simulink model "TOGGLER"  (R2022b)
settings: Solver=FixedStepDiscrete  StartTime=0  StopTime=duration  FixedStep=sample_time  RelTol=1e-3
values from neighbouring files (symbols this model uses):
  CTRL =     [TOGGLER_params.mat]
  CTRLSector =     [TOGGLER_params.mat]
  Greedy_Status = 1    [TOGGLER_params.mat]    (also in init_TOGGLER.m = logical(true))
  sample_time = 0.1    [TOGGLER_params.mat]
  WFC_1_Status = 1    [TOGGLER_params.mat]    (also in init_TOGGLER.m = logical(true))
  WFC_2_Status = 1    [TOGGLER_params.mat]    (also in init_TOGGLER.m = logical(true))
  WFC_3_Status = 1    [TOGGLER_params.mat]    (also in init_TOGGLER.m = logical(true))
undefined symbols (not defined in the file or in its folder): j
libraries: simulink x39, dspindex x14, dspstat3 x4, dspsigops x1
(part 1 of 2)
settings Model: Creator=Carlo_TUM  LastModifiedBy=Carlo_TUM
settings DataIOCC: LoadExternalInput=on  ReturnWorkspaceOutputs=off  ReturnWorkspaceOutputsName=off
settings OptimizationCC: DefaultParameterBehavior=Inlined  EnhancedBackFolding=on  PassReuseOutputArgsAs=Individual arguments  OptimizeBlockOrder=speed  DifferentSizesBufferReuse=on  OptimizationCustomize=off  EfficientTunableParamExpr=on
settings DebuggingCC: ParameterTunabilityLossMsg=error
settings SFSimCC: MATLABDynamicMemAlloc=off
settings RTWCC: Description=Embedded Coder  SystemTargetFile=ert.tlc  TemplateMakefile=ert_default_tmf
settings CodeAppCC: ForceParamTrailComments=on  IgnoreCustomStorageClasses=off  OperatorAnnotations=on  SimulinkDataObjDesc=on  SFDataObjDesc=on  InsertBlockDesc=on
settings ERTTargetCC: GenerateSampleERTMain=on  InlinedParameterPlacement=NonHierarchical  ERTCustomFileTemplate=example_file_process.tlc

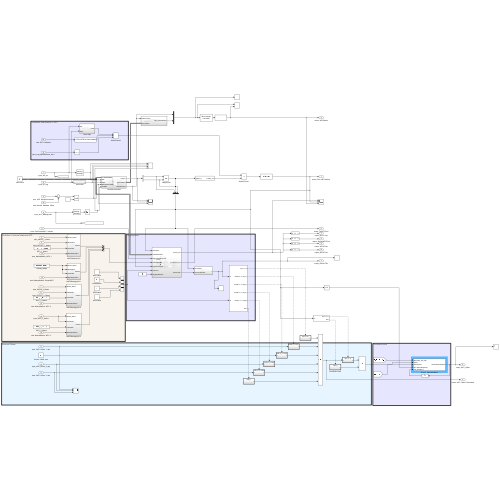
[thumbnail: Simulink's stored preview of the top-level diagram]
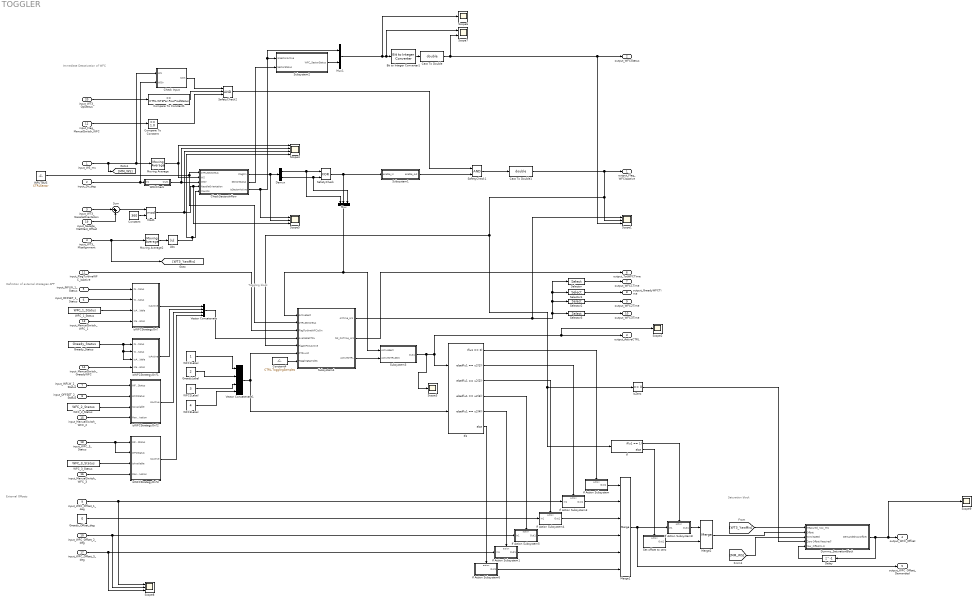
== system TOGGLER ==
  note: Definition of external strategies APP
  note: Toggling block
  note: External Offsets
  note: Saturation block
  note: Immediate Deactivation of WFC
  input_WS_ms : Inport  PortDimensions=1
  input_Dir_deg : Inport  Port=2  PortDimensions=1
  input_WT3_NacelleOrientation : Inport  Port=3  OutDataTypeStr=double  PortDimensions=1
  input_WT3_Misalignment : Inport  Port=4  OutDataTypeStr=double  PortDimensions=1
  input_INFLW_1_Status : Inport  Port=5  OutDataTypeStr=double
  input_OFFSET_1_Status : Inport  Port=6  OutDataTypeStr=double
  input_INFLW_2_Status : Inport  Port=7  OutDataTypeStr=double
  input_OFFSET_2_Status : Inport  Port=8
  input_WFC_Offset_1_deg : Inport  Port=9
  input_WFC_Offset_2_deg : Inport  Port=10
  input_FlagTurbineWFC_isActive : Inport  Port=11
  input_Flag_ManualSwitch_WFC : Inport  Port=12  PortDimensions=1
  input_ManualSwitch_WFC_1 : Inport  Port=13  PortDimensions=1
  input_ManualSwitch_GreedyWFC : Inport  Port=14  PortDimensions=1
  input_ManualSwitch_WFC_2 : Inport  Port=15  PortDimensions=1
  input_ManualSwitch_WFC_3 : Inport  Port=16  PortDimensions=1
  input_WFC_Offset_3_deg : Inport  Port=17  PortDimensions=1
  input_WFC_3_Status : Inport  Port=18  PortDimensions=1
  input_Nacelle_MetMast_Offset : Inport  Port=19  PortDimensions=1
  input_WT3_OpStatus : Inport  Port=20  PortDimensions=1
  Abs : Abs  SaturateOnIntegerOverflow=off
  Bit to Integer Converter1 : simulink/Logic and Bit Operations/Bit to Integer Converter  nbits=5  bitOrder=MSB first  signedOutputValues=Unsigned  outDtype=Inherit via internal rule  outDtypeSigned=Inherit via internal rule
      settings: LibrarySourceBlock=|
      | commutil2/Bit to Integer
      | Converter
  Cast To Double : DataTypeConversion  OutDataTypeStr=double  SaturateOnIntegerOverflow=off  RndMeth=Floor
  Cast To Double1 : DataTypeConversion  OutDataTypeStr=double  SaturateOnIntegerOverflow=off  RndMeth=Floor
  Check Input : Subsystem
  CheckSectorsInflow : Subsystem
  Compare To Constant : simulink/Logic and Bit Operations/Compare To Constant  relop===  const=1.0  OutDataTypeStr=boolean
  Compare To Constant1 : simulink/Logic and Bit Operations/Compare To Constant  relop===  const=CTRL.WT3Par.PowProdStatus  OutDataTypeStr=boolean
  Constant : Constant  Value=360
  Constant4 : Constant  Value=CTRL.TogglingSamples
  Delay : Delay  DelayLength=1  InitialCondition=0
  Demux : Demux  Outputs=2
  Dummy_SaturationBlock : Subsystem
  GreedyLabel : Constant  Value=2
  Greedy_Offset_deg : Constant  Value=0  OutDataTypeStr=Inherit: Inherit via back propagation
  Greedy_Status : Constant  Value=Greedy_Status
  INPUTBUS : Constant  Value=CTRLSector  VectorParams1D=off  OutDataTypeStr=Bus: CTRLSector_Bus
  If : If  IfExpression=u1 == 1
  If Action Subsystem : Subsystem  TreatAsAtomicUnit=on
  If Action Subsystem1 : Subsystem  TreatAsAtomicUnit=on
  If Action Subsystem3 : Subsystem  TreatAsAtomicUnit=on
  If Action Subsystem4 : Subsystem  TreatAsAtomicUnit=on
  If Action Subsystem5 : Subsystem  TreatAsAtomicUnit=on
  If Action Subsystem6 : Subsystem  TreatAsAtomicUnit=on
  If Action Subsystem8 : Subsystem  TreatAsAtomicUnit=on
  If3 : If  NumInputs=2  IfExpression=u1 == 0  ElseIfExpressions=u1 == u2(1) , u1 == u2(2) , u1 == u2(3) , u1 == u2(4)
  IsZero : simulink/Logic and Bit Operations/Compare To Zero  relop===  OutDataTypeStr=boolean
  Merge1 : Merge  Inputs=6
  Merge2 : Merge
  Mod1 : Math  Operator=mod  SignedPower=on
  Moving Average : dspstat3/Moving Average  Method=Sliding window  ForgettingFactorPort=off  SpecifyWindowLength=on  WindowLength=CTRL.MovAvWS  OverlapLength=CTRL.MovAvWS - 1  AllowArbitraryInputLength=off  ForgettingFactor=0.9  SimulateUsing=Code generation
  Moving Average2 : dspstat3/Moving Average  Method=Sliding window  ForgettingFactorPort=off  SpecifyWindowLength=on  WindowLength=CTRL.MovAvWMisalignment  OverlapLength=CTRL.MovAvWMisalignment - 1  AllowArbitraryInputLength=off  ForgettingFactor=0.9  SimulateUsing=Code generation
  Mux : Mux  Inputs=3
  Mux1 : Mux  Inputs=2
  SafetyCheck : Logic  Operator=XOR  AllPortsSameDT=off  OutDataTypeStr=boolean
  SafetyCheck1 : Logic  AllPortsSameDT=off  OutDataTypeStr=boolean
  SafetyCheck2 : Logic  Inputs=3  AllPortsSameDT=off  OutDataTypeStr=boolean
  Scope1 : Scope  NumInputPorts=3
  Scope{2..3,6,9} (4 alike) : Scope
  Scope4 : Scope  NumInputPorts=4
  Scope5 : Scope  NumInputPorts=3
  Scope7 : Scope  NumInputPorts=2
  Scope8 : Scope  NumInputPorts=3
  Selector : Selector  InputPortWidth=4  IndexOptions=Index vector (dialog)  Indices=[1]  OutputSizes=1
  Selector1 : Selector  InputPortWidth=4  IndexOptions=Index vector (dialog)  Indices=[2]  OutputSizes=1
  Selector2 : Selector  InputPortWidth=4  IndexOptions=Index vector (dialog)  Indices=[3]  OutputSizes=1
  Selector3 : Selector  InputPortWidth=4  IndexOptions=Index vector (dialog)  Indices=[4]  OutputSizes=1
  Set offset to zero : Subsystem  TreatAsAtomicUnit=on
  Subsystem1 : Subsystem  mask(Signal holding){wait_time=CTRL.InflowChecks_WaitTime, sampling_time=sample_time, selection=off}
      mask prompts: wait_time "Wait time [s]"; sampling_time "Sampling time [s]"; selection "Instant disabling"
      mask help:
      | The block prevents fast switching of the input signal. After the input is changed, it waits for the defined time before changing the output, if the input doesn't change within this period, the output is switched.
      | The option "Instant disabling" only enforces waiting time on rising edge, but always allows the signal to go to zero.
      | Ask Vlaho for help.
      mask init:
      | Counter = wait_time/sampling_time;
      mask Help:
      | No documentation, ask Vlaho for help. ;)
      | 22 Nov 2020
  Subsystem2 : Subsystem
  Subsystem3 : Subsystem
  Subsystem4 : Subsystem
  Sum : Sum  Inputs=|++
  Vector Concatenate : Concatenate  NumInputs=4
  Vector Concatenate1 : Concatenate  NumInputs=4
  WDirCheck : Subsystem
  WFC1Label : Constant
  WFC2Label : Constant  Value=3
  WFC3Label : Constant  Value=4
  WFC_1_Status : Constant  Value=WFC_1_Status
  WFC_2_Status : Constant  Value=WFC_2_Status
  WFC_3_Status : Constant  Value=WFC_3_Status
  isWFCStrategyOn? : Subsystem
  isWFCStrategyOn?1 : Subsystem
  isWFCStrategyOn?2 : Subsystem
  isWFCStrategyOn?3 : Subsystem
  output_Flag_WFCIsActive : Outport  VectorParamsAs1DForOutWhenUnconnected=off
  output_WFCStatus : Outport  Port=2  VectorParamsAs1DForOutWhenUnconnected=off
  output_ActiveCTRL : Outport  Port=3  VectorParamsAs1DForOutWhenUnconnected=off
  output_WFC_Offset : Outport  Port=4  VectorParamsAs1DForOutWhenUnconnected=off
  output_WFC_Offset_Demanded : Outport  Port=5  VectorParamsAs1DForOutWhenUnconnected=off
  output_TotWFCTime : Outport  Port=6  VectorParamsAs1DForOutWhenUnconnected=off
  output_WFC1Time : Outport  Port=7  VectorParamsAs1DForOutWhenUnconnected=off
  output_GreedyWFCTime : Outport  Port=8  VectorParamsAs1DForOutWhenUnconnected=off
  output_WFC2Time : Outport  Port=9  VectorParamsAs1DForOutWhenUnconnected=off
  output_WFC3Time : Outport  Port=10  VectorParamsAs1DForOutWhenUnconnected=off
  wires:
  SafetyCheck1/1 -> Cast To Double1/1
  Subsystem4/3(ActiveCTRL) -> Subsystem3/2(ActiveCTRLSect)
  If3/1 -> If Action Subsystem/Action
  Abs/1 -> CheckSectorsInflow/5(YawMis), Scope4/4
  CheckSectorsInflow/2(SectorStatus) -> Subsystem2/2(SectorStatus)
  input_ManualSwitch_GreedyWFC/1 -> isWFCStrategyOn?1/4(ManualActivation)
  input_Dir_deg/1 -> Check Input/2(WDir), WDirCheck/1(In1)
  Selector3/1 -> output_WFC3Time/1
  isWFCStrategyOn?2/1(isActive) -> Vector Concatenate/3
  Vector Concatenate1/1 -> Subsystem4/6(CTRLList), If3/2
  input_ManualSwitch_WFC_1/1 -> isWFCStrategyOn?/4(ManualActivation)
  Demux/1 -> Mux/1, SafetyCheck/1
  Selector1/1 -> output_GreedyWFCTime/1
  Dummy_SaturationBlock/1(DemandedYawOffset) -> Delay/1, Scope9/1, output_WFC_Offset/1
  input_WS_ms/1 -> Check Input/1(WS), Moving Average/1, [MM_WS]
  input_Nacelle_MetMast_Offset/1 -> Sum/2
  Check Input/1(IsOK) -> SafetyCheck2/1
  WFC_1_Status/1 -> isWFCStrategyOn?/3(isAvailable)
  input_INFLW_2_Status/1 -> isWFCStrategyOn?2/1(INFLW_Status)
  input_Flag_ManualSwitch_WFC/1 -> Compare To Constant/1
  isWFCStrategyOn?/1(isActive) -> Vector Concatenate/1
  SafetyCheck/1 -> Subsystem1/1(enable_in), Mux/2
  Compare To Constant1/1 -> SafetyCheck2/2
  input_WT3_OpStatus/1 -> Compare To Constant1/1
  If Action Subsystem1/1(Out1) -> Merge1/5
  If Action Subsystem5/1(Out1) -> Merge1/4
  [WT3_YawMis] -> Dummy_SaturationBlock/1(Measured_Yaw_Mis)
  input_WT3_Misalignment/1 -> [WT3_YawMis], Moving Average2/1
  input_WFC_3_Status/1 -> isWFCStrategyOn?3/2(WFCStatus), isWFCStrategyOn?3/1(INFLW_Status)
  WFC_3_Status/1 -> isWFCStrategyOn?3/3(isAvailable)
  Constant/1 -> Mod1/2
  isWFCStrategyOn?3/1(isActive) -> Vector Concatenate/4
  input_WFC_Offset_1_deg/1 -> Scope8/1, If Action Subsystem3/1(In1)
  Delay/1 -> Dummy_SaturationBlock/5(Yaw_Offset(k-1))
  WFC3Label/1 -> Vector Concatenate1/4
  If3/5 -> If Action Subsystem1/Action
  CheckSectorsInflow/3(isSectorActive) -> Scope5/1, Mux1/1, Subsystem2/1(isSectorActive)
  Greedy_Status/1 -> isWFCStrategyOn?1/2(WFCStatus), isWFCStrategyOn?1/3(isAvailable), isWFCStrategyOn?1/1(INFLW_Status)
  Constant4/1 -> Subsystem4/7(TogglingSamples)
  If3/3 -> If Action Subsystem4/Action
  Cast To Double1/1 -> IsZero/1, If/1, Subsystem4/5(FlagWFCIsActive), Scope1/2, output_Flag_WFCIsActive/1
  Subsystem4/2(tot_OnTime_Hrs) -> output_TotWFCTime/1
  Subsystem4/1(onTime_Hrs) -> Scope1/1, Selector3/1, Selector/1, Selector1/1, Selector2/1
  isWFCStrategyOn?1/1(isActive) -> Vector Concatenate/2
  If Action Subsystem4/1(Out1) -> Merge1/3
  input_ManualSwitch_WFC_2/1 -> isWFCStrategyOn?2/4(ManualActivation)
  input_FlagTurbineWFC_isActive/1 -> Subsystem4/3(FlagTurbineWFCIsOn)
  Vector Concatenate/1 -> Subsystem4/4(AvailableCTRL)
  Selector2/1 -> output_WFC2Time/1
  If Action Subsystem8/1(Out1) -> Merge2/1
  GreedyLabel/1 -> Vector Concatenate1/2
  WFC_2_Status/1 -> isWFCStrategyOn?2/3(isAvailable)
  SafetyCheck2/1 -> SafetyCheck1/1
  input_ManualSwitch_WFC_3/1 -> isWFCStrategyOn?3/4(ManualActivation)
  input_OFFSET_1_Status/1 -> isWFCStrategyOn?/2(WFCStatus)
  Subsystem3/1(Out1) -> Scope3/1, output_ActiveCTRL/1, Scope2/1, If3/1
  INPUTBUS/1 -> Subsystem4/2(CTRLSectorBus), CheckSectorsInflow/1(CTRLSectorBus)
  Merge1/1 -> output_WFC_Offset_Demanded/1, If Action Subsystem8/1(In1)
  IsZero/1 -> Dummy_SaturationBlock/4(Zero Offset Required?)
  Mod1/1 -> Scope5/3, CheckSectorsInflow/4(NacelleOrientation), Scope4/3
  input_OFFSET_2_Status/1 -> isWFCStrategyOn?2/2(WFCStatus)
  input_WFC_Offset_3_deg/1 -> Scope8/3, If Action Subsystem1/1(In1)
  input_WFC_Offset_2_deg/1 -> Scope8/2, If Action Subsystem5/1(In1)
  Moving Average/1 -> CheckSectorsInflow/2(WS), Scope4/1
  Mux1/1 -> Scope6/1, Scope7/1, Bit to Integer Converter1/1
  WDirCheck/1(Out1) -> Scope4/2, CheckSectorsInflow/3(WDir)
  input_WT3_NacelleOrientation/1 -> Sum/1
  Merge2/1 -> Dummy_SaturationBlock/2(Offset)
  Mux/1 -> Subsystem3/1(ActiveSect), Subsystem4/1(ActiveSect)
  Cast To Double/1 -> Scope7/2, Scope1/3, output_WFCStatus/1
  CheckSectorsInflow/1(FlagOn) -> Scope5/2, Demux/1
  Sum/1 -> Mod1/1
  Bit to Integer Converter1/1 -> Cast To Double/1
  [MM_WS] -> Dummy_SaturationBlock/3(Wind Speed)
  input_INFLW_1_Status/1 -> isWFCStrategyOn?/1(INFLW_Status)
  Selector/1 -> output_WFC1Time/1
  WFC2Label/1 -> Vector Concatenate1/3
  Subsystem1/1(enable_out) -> SafetyCheck1/2
  Demux/2 -> Mux/3, SafetyCheck/2
  If3/2 -> If Action Subsystem3/Action
  If/2 -> Set offset to zero/Action
  WFC1Label/1 -> Vector Concatenate1/1
  Moving Average2/1 -> Abs/1
  Subsystem2/1(WFC_SectorStatus) -> Mux1/2
  Set offset to zero/1(Out1) -> Merge2/2
  Compare To Constant/1 -> SafetyCheck2/3
  If3/6 -> If Action Subsystem6/Action
  If3/4 -> If Action Subsystem5/Action
  Greedy_Offset_deg/1 -> If Action Subsystem4/1(In1)
  If Action Subsystem/1(Out1) -> Merge1/1
  If Action Subsystem6/1(Out1) -> Merge1/6
  If Action Subsystem3/1(Out1) -> Merge1/2
  If/1 -> If Action Subsystem8/Action

== system TOGGLER/Check Input ==
  WS : Inport
  WDir : Inport  Port=2
  Constant2 : Constant  Value=CTRL.InputCheck.StartupTimeSamples
  Logical Operator : Logic  Operator=OR  AllPortsSameDT=off  OutDataTypeStr=boolean
  NOT : Logic  Operator=NOT  IconShape=distinctive  AllPortsSameDT=off  OutDataTypeStr=boolean
  Scope9 : Scope  NumInputPorts=2
  Subsystem5 : Subsystem
  Subsystem6 : Subsystem
  Terminator : Terminator
  Terminator1 : Terminator
  IsOK : Outport  VectorParamsAs1DForOutWhenUnconnected=off
  wires:
  Subsystem6/1(Var) -> Terminator/1
  Subsystem5/1(Var) -> Terminator1/1
  Constant2/1 -> Subsystem6/2(StartupTimeSamples), Subsystem5/2(StartupTimeSamples)
  WS/1 -> Subsystem6/1(InVar)
  Subsystem6/2(ErrorFlag) -> Logical Operator/1, Scope9/1
  Subsystem5/2(ErrorFlag) -> Logical Operator/2, Scope9/2
  WDir/1 -> Subsystem5/1(InVar)
  Logical Operator/1 -> NOT/1
  NOT/1 -> IsOK/1

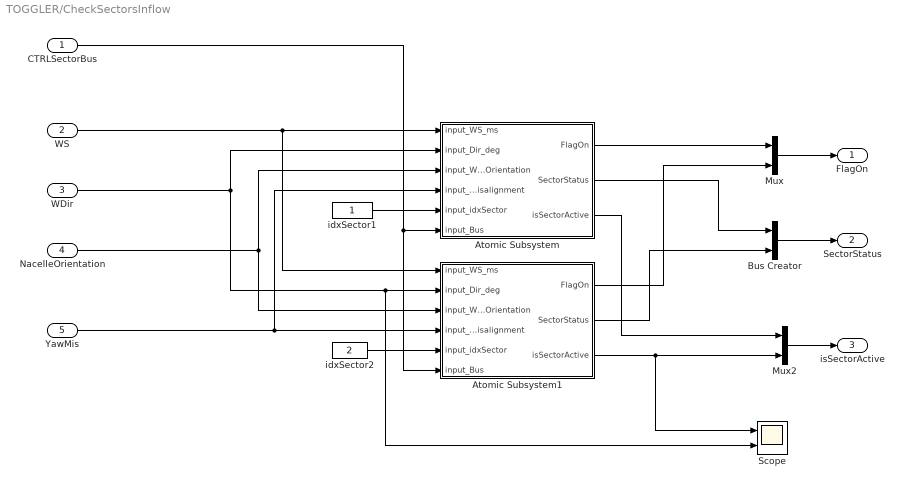
== system TOGGLER/CheckSectorsInflow ==
  CTRLSectorBus : Inport  OutDataTypeStr=Bus: CTRLSector_Bus
  WS : Inport  Port=2
  WDir : Inport  Port=3
  NacelleOrientation : Inport  Port=4
  YawMis : Inport  Port=5
  Atomic Subsystem : Subsystem  TreatAsAtomicUnit=on
  Atomic Subsystem1 : Subsystem  TreatAsAtomicUnit=on
  Bus Creator : BusCreator  Inputs=2
  Mux : Mux  Inputs=2
  Mux2 : Mux  Inputs=2
  Scope : Scope  NumInputPorts=2
  idxSector1 : Constant
  idxSector2 : Constant  Value=2
  FlagOn : Outport  VectorParamsAs1DForOutWhenUnconnected=off
  SectorStatus : Outport  Port=2  VectorParamsAs1DForOutWhenUnconnected=off
  isSectorActive : Outport  Port=3  VectorParamsAs1DForOutWhenUnconnected=off
  wires:
  Atomic Subsystem1/1(FlagOn) -> Mux/2
  idxSector1/1 -> Atomic Subsystem/5(input_idxSector)
  idxSector2/1 -> Atomic Subsystem1/5(input_idxSector)
  YawMis/1 -> Atomic Subsystem/4(input_WT3_Misalignment), Atomic Subsystem1/4(input_WT3_Misalignment)
  WS/1 -> Atomic Subsystem1/1(input_WS_ms), Atomic Subsystem/1(input_WS_ms)
  NacelleOrientation/1 -> Atomic Subsystem/3(input_WT3_NacelleOrientation), Atomic Subsystem1/3(input_WT3_NacelleOrientation)
  CTRLSectorBus/1 -> Atomic Subsystem1/6(input_Bus), Atomic Subsystem/6(input_Bus)
  WDir/1 -> Atomic Subsystem/2(input_Dir_deg), Scope/2, Atomic Subsystem1/2(input_Dir_deg)
  Atomic Subsystem/2(SectorStatus) -> Bus Creator/1
  Atomic Subsystem1/2(SectorStatus) -> Bus Creator/2
  Atomic Subsystem/3(isSectorActive) -> Mux2/1
  Atomic Subsystem1/3(isSectorActive) -> Scope/1, Mux2/2
  Atomic Subsystem/1(FlagOn) -> Mux/1
  Mux/1 -> FlagOn/1
  Bus Creator/1 -> SectorStatus/1
  Mux2/1 -> isSectorActive/1

== system TOGGLER/Dummy_SaturationBlock ==
  note: This is a dummy saturation block. In a real case, this block should include the actual control logic of the WT to prevent unwanted shut down during WFC
  Measured_Yaw_Mis : Inport
  Offset : Inport  Port=2
  Wind Speed : Inport  Port=3
  Zero Offset Required? : Inport  Port=4
  Yaw_Offset(k-1) : Inport  Port=5
  Saturation : Saturate  UpperLimit=CTRL.SatBlock.WFC_OffsetRange(2)  LowerLimit=CTRL.SatBlock.WFC_OffsetRange(1)
  Terminator{,1..2,4} (4 alike) : Terminator
  DemandedYawOffset : Outport  PortDimensions=1
  wires:
  Offset/1 -> Saturation/1
  Saturation/1 -> DemandedYawOffset/1
  Wind Speed/1 -> Terminator1/1
  Zero Offset Required?/1 -> Terminator/1
  Yaw_Offset(k-1)/1 -> Terminator2/1
  Measured_Yaw_Mis/1 -> Terminator4/1

== system TOGGLER/If Action Subsystem ==
  Action Port : ActionPort  ActionPortLabel=if(u1 == 0)
  Zero : Constant  Value=0  OutDataTypeStr=Inherit: Inherit via back propagation
  Out1 : Outport  VectorParamsAs1DForOutWhenUnconnected=off
  wires:
  Zero/1 -> Out1/1

== system TOGGLER/If Action Subsystem1 ==
  In1 : Inport
  Action Port : ActionPort  ActionPortLabel=elseif( u1 == u2(4))
  Out1 : Outport  VectorParamsAs1DForOutWhenUnconnected=off
  wires:
  In1/1 -> Out1/1

== system TOGGLER/If Action Subsystem3 ==
  In1 : Inport
  Action Port : ActionPort  ActionPortLabel=elseif(u1 == u2(1) )
  Out1 : Outport  VectorParamsAs1DForOutWhenUnconnected=off
  wires:
  In1/1 -> Out1/1

== system TOGGLER/If Action Subsystem4 ==
  In1 : Inport
  Action Port : ActionPort  ActionPortLabel=elseif( u1 == u2(2) )
  Out1 : Outport  VectorParamsAs1DForOutWhenUnconnected=off
  wires:
  In1/1 -> Out1/1

== system TOGGLER/If Action Subsystem5 ==
  In1 : Inport
  Action Port : ActionPort  ActionPortLabel=elseif( u1 == u2(3) )
  Out1 : Outport  VectorParamsAs1DForOutWhenUnconnected=off
  wires:
  In1/1 -> Out1/1

== system TOGGLER/If Action Subsystem6 ==
  Action Port : ActionPort  ActionPortLabel=else
  Zero : Constant  Value=0  OutDataTypeStr=Inherit: Inherit via back propagation
  Out1 : Outport  VectorParamsAs1DForOutWhenUnconnected=off
  wires:
  Zero/1 -> Out1/1

== system TOGGLER/If Action Subsystem8 ==
  In1 : Inport
  Action Port : ActionPort  ActionPortLabel=if(u1 == 1)
  Out1 : Outport  VectorParamsAs1DForOutWhenUnconnected=off
  wires:
  In1/1 -> Out1/1

== system TOGGLER/Set offset to zero ==
  Action Port : ActionPort  ActionPortLabel=else
  Zero : Constant  Value=0  OutDataTypeStr=Inherit: Inherit via back propagation
  Out1 : Outport  VectorParamsAs1DForOutWhenUnconnected=off
  wires:
  Zero/1 -> Out1/1

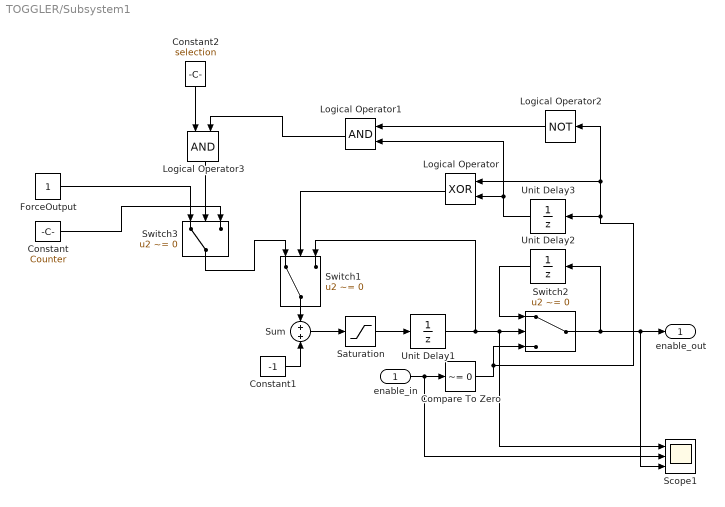
== system TOGGLER/Subsystem1 ==
  enable_in : Inport
  Compare To Zero : simulink/Logic and Bit Operations/Compare To Zero  relop=~=  OutDataTypeStr=boolean
  Constant : Constant  Value=Counter
  Constant1 : Constant  Value=-1
  Constant2 : Constant  Value=selection
  ForceOutput : Constant  OutDataTypeStr=Inherit: Inherit via back propagation
  Logical Operator : Logic  Operator=XOR  AllPortsSameDT=off  OutDataTypeStr=boolean
  Logical Operator1 : Logic  AllPortsSameDT=off  OutDataTypeStr=boolean
  Logical Operator2 : Logic  Operator=NOT  AllPortsSameDT=off  OutDataTypeStr=boolean
  Logical Operator3 : Logic  AllPortsSameDT=off  OutDataTypeStr=boolean
  Saturation : Saturate  UpperLimit=inf  LowerLimit=-inf
  Scope1 : Scope  NumInputPorts=3
  Sum : Sum
  Switch1 : Switch  Criteria=u2 ~= 0  SaturateOnIntegerOverflow=off  InputSameDT=off
  Switch2 : Switch  Criteria=u2 ~= 0  SaturateOnIntegerOverflow=off  InputSameDT=off
  Switch3 : Switch  Criteria=u2 ~= 0  SaturateOnIntegerOverflow=off  InputSameDT=off
  Unit Delay1 : UnitDelay  SampleTime=sampling_time  HasFrameUpgradeWarning=on
  Unit Delay2 : UnitDelay  SampleTime=sampling_time  HasFrameUpgradeWarning=on
  Unit Delay3 : UnitDelay  SampleTime=sampling_time  HasFrameUpgradeWarning=on
  enable_out : Outport
  wires:
  Saturation/1 -> Unit Delay1/1
  Unit Delay2/1 -> Switch2/1
  Switch2/1 -> Scope1/3, enable_out/1, Unit Delay2/1
  Sum/1 -> Saturation/1
  Switch1/1 -> Sum/1
  Constant1/1 -> Sum/2
  Constant/1 -> Switch3/3
  Logical Operator/1 -> Switch1/2
  enable_in/1 -> Scope1/2, Compare To Zero/1
  Logical Operator2/1 -> Logical Operator1/1
  Logical Operator1/1 -> Logical Operator3/2
  Compare To Zero/1 -> Switch2/3, Unit Delay3/1, Logical Operator/1, Logical Operator2/1
  Unit Delay3/1 -> Logical Operator/2, Logical Operator1/2
  Unit Delay1/1 -> Switch1/3, Scope1/1, Switch2/2
  Constant2/1 -> Logical Operator3/1
  ForceOutput/1 -> Switch3/1
  Switch3/1 -> Switch1/1
  Logical Operator3/1 -> Switch3/2

== system TOGGLER/Subsystem2 ==
  isSectorActive : Inport
  SectorStatus : Inport  Port=2
  Bus Selector : BusSelector  OutputSignals=signal1,signal2
  Demux : Demux  Outputs=2
  Enabled Subsystem : Subsystem  TreatAsAtomicUnit=on
  Enabled Subsystem1 : Subsystem  TreatAsAtomicUnit=on
  Gain : Gain  Gain=0
  Logical Operator : Logic  Operator=XOR  AllPortsSameDT=off  OutDataTypeStr=boolean
  Merge3 : Merge
  Switch : Switch  Criteria=u2 ~= 0  SaturateOnIntegerOverflow=off  InputSameDT=off
  WFC_SectorStatus : Outport  VectorParamsAs1DForOutWhenUnconnected=off
  wires:
  Demux/1 -> Logical Operator/1, Enabled Subsystem/Enable
  Logical Operator/1 -> Switch/2
  Bus Selector/2 -> Enabled Subsystem1/1(In1)  "<signal2>"
  Enabled Subsystem/1(Out1) -> Merge3/1
  Gain/1 -> Switch/3
  Merge3/1 -> Switch/1
  Bus Selector/1 -> Gain/1, Enabled Subsystem/1(In1)  "<signal1>"
  Enabled Subsystem1/1(Out1) -> Merge3/2
  Demux/2 -> Logical Operator/2, Enabled Subsystem1/Enable
  SectorStatus/1 -> Bus Selector/1
  Switch/1 -> WFC_SectorStatus/1
  isSectorActive/1 -> Demux/1

== system TOGGLER/Subsystem3 ==
  ActiveSect : Inport
  ActiveCTRLSect : Inport  Port=2
  Demux1 : Demux  Outputs=3
  Demux2 : Demux  Outputs=2
  Enabled Subsystem : Subsystem  TreatAsAtomicUnit=on
  Enabled Subsystem1 : Subsystem  TreatAsAtomicUnit=on
  Enabled Subsystem2 : Subsystem  TreatAsAtomicUnit=on
  Enabled Subsystem3 : Subsystem  TreatAsAtomicUnit=on
  Merge : Merge  Inputs=3
  Subsystem : Subsystem
  Out1 : Outport  VectorParamsAs1DForOutWhenUnconnected=off
  wires:
  Demux2/2 -> Enabled Subsystem2/4(ActiveCTRL_S2), Enabled Subsystem1/1(In1)
  ActiveSect/1 -> Demux1/1
  Demux1/2 -> Subsystem/2(XOR)
  Subsystem/3(Off) -> Enabled Subsystem3/Enable
  Demux1/1 -> Subsystem/1(Sect1)
  Demux1/3 -> Subsystem/3(Sect2)
  ActiveCTRLSect/1 -> Demux2/1
  Subsystem/2(Sector2_Flag) -> Enabled Subsystem1/Enable, Enabled Subsystem2/2(Sector2_Flag)
  Subsystem/1(Sector1_Flag) -> Enabled Subsystem/Enable, Enabled Subsystem2/1(Sector1_Flag)
  Demux2/1 -> Enabled Subsystem2/3(ActiveCTRL_S1), Enabled Subsystem/1(In1)
  Enabled Subsystem/1(Out1) -> Merge/2
  Enabled Subsystem1/1(Out1) -> Merge/3
  Enabled Subsystem2/1(Out1) -> Enabled Subsystem3/1(In1)
  Merge/1 -> Out1/1
  Enabled Subsystem3/1(Out1) -> Merge/1

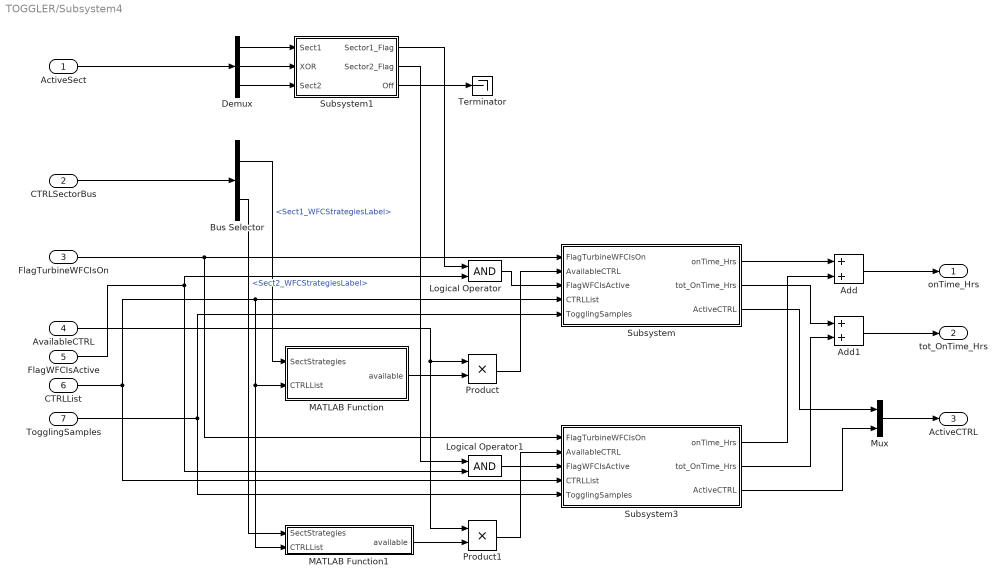
== system TOGGLER/Subsystem4 ==
  ActiveSect : Inport
  CTRLSectorBus : Inport  Port=2  OutDataTypeStr=Bus: CTRLSector_Bus
  FlagTurbineWFCIsOn : Inport  Port=3
  AvailableCTRL : Inport  Port=4
  FlagWFCIsActive : Inport  Port=5
  CTRLList : Inport  Port=6
  TogglingSamples : Inport  Port=7
  Add : Sum
  Add1 : Sum
  Bus Selector : BusSelector  OutputSignals=Sect1_WFCStrategiesLabel,Sect2_WFCStrategiesLabel
  Demux : Demux  Outputs=3
  Logical Operator : Logic  AllPortsSameDT=off  OutDataTypeStr=boolean
  Logical Operator1 : Logic  AllPortsSameDT=off  OutDataTypeStr=boolean
  MATLAB Function : MATLAB Function  TreatAsAtomicUnit=on
  MATLAB Function1 : MATLAB Function  TreatAsAtomicUnit=on
  Mux : Mux  Inputs=2
  Product : Product
  Product1 : Product
  Subsystem : Subsystem
  Subsystem1 : Subsystem
  Subsystem3 : Subsystem
  Terminator : Terminator
  onTime_Hrs : Outport  VectorParamsAs1DForOutWhenUnconnected=off
  tot_OnTime_Hrs : Outport  Port=2  VectorParamsAs1DForOutWhenUnconnected=off
  ActiveCTRL : Outport  Port=3  VectorParamsAs1DForOutWhenUnconnected=off
  wires:
  CTRLSectorBus/1 -> Bus Selector/1
  FlagTurbineWFCIsOn/1 -> Subsystem3/1(FlagTurbineWFCIsOn), Subsystem/1(FlagTurbineWFCIsOn)
  FlagWFCIsActive/1 -> Logical Operator1/2, Logical Operator/2
  CTRLList/1 -> Subsystem3/4(CTRLList), MATLAB Function1/2(CTRLList), MATLAB Function/2(CTRLList), Subsystem/4(CTRLList)
  TogglingSamples/1 -> Subsystem3/5(TogglingSamples), Subsystem/5(TogglingSamples)
  Bus Selector/1 -> MATLAB Function/1(SectStrategies)  "<Sect1_WFCStrategiesLabel>"
  MATLAB Function/1(available) -> Product/2
  Bus Selector/2 -> MATLAB Function1/1(SectStrategies)  "<Sect2_WFCStrategiesLabel>"
  MATLAB Function1/1(available) -> Product1/2
  AvailableCTRL/1 -> Product1/1, Product/1
  Product/1 -> Subsystem/2(AvailableCTRL)
  Product1/1 -> Subsystem3/2(AvailableCTRL)
  Subsystem/1(onTime_Hrs) -> Add/1
  Subsystem3/1(onTime_Hrs) -> Add/2
  Subsystem/2(tot_OnTime_Hrs) -> Add1/1
  Subsystem3/2(tot_OnTime_Hrs) -> Add1/2
  Add/1 -> onTime_Hrs/1
  Add1/1 -> tot_OnTime_Hrs/1
  Subsystem/3(ActiveCTRL) -> Mux/1
  Subsystem3/3(ActiveCTRL) -> Mux/2
  Mux/1 -> ActiveCTRL/1
  ActiveSect/1 -> Demux/1
  Demux/1 -> Subsystem1/1(Sect1)
  Demux/2 -> Subsystem1/2(XOR)
  Demux/3 -> Subsystem1/3(Sect2)
  Subsystem1/1(Sector1_Flag) -> Logical Operator/1
  Logical Operator/1 -> Subsystem/3(FlagWFCIsActive)
  Subsystem1/2(Sector2_Flag) -> Logical Operator1/1
  Logical Operator1/1 -> Subsystem3/3(FlagWFCIsActive)
  Subsystem1/3(Off) -> Terminator/1

== system TOGGLER/WDirCheck ==
  In1 : Inport
  Compare To Constant : simulink/Logic and Bit Operations/Compare To Constant  relop=>=  const=600.0  OutDataTypeStr=boolean
  Delay : Delay  DelayLength=1  InitialCondition=0
  Ground : Ground
  Sample and Hold : dspsigops/Sample and Hold  trig=Rising edge  initCond=0  latchinput=off
  Scope : Scope  NumInputPorts=3
  Subsystem5 : Subsystem  mask(Moving average & standard deviation for angles){filt_T=CTRL.MovAvWDir*sample_time, filt_wait=CTRL.MovAvWDir*sample_time, sample_time=sample_time}
      mask prompts: filt_T "Window duration"; filt_wait "Waiting time before providing output"; sample_time "Sample time"
      mask help:
      | Computes moving average and standard deviation for angular values in degrees over a time window. All parameters are expressed in seconds.
      | Ask Vlaho for details.
      | 25 Nov 2020
      mask init:
      | N_filt = ceil(filt_T / sample_time);
      | if N_filt<1, N_filt = 1; end
      | lower_limit = ceil(filt_wait / sample_time);
      | if lower_limit<2, lower_limit = 2; end
      mask Help: No help provided, ask Vlaho for details. ;)
  Switch : Switch  Criteria=u2 ~= 0  SaturateOnIntegerOverflow=off  InputSameDT=off
  Terminator : Terminator
  Terminator1 : Terminator
  Terminator2 : Terminator
  Out1 : Outport  VectorParamsAs1DForOutWhenUnconnected=off
  wires:
  Subsystem5/4(output_OK) -> Terminator2/1
  Ground/1 -> Subsystem5/2(reset)
  In1/1 -> Switch/3, Compare To Constant/1, Delay/1
  Subsystem5/2(std [deg]) -> Terminator/1
  Subsystem5/1(mean [deg]) -> Scope/2, Out1/1
  Subsystem5/3(window_length) -> Terminator1/1
  Compare To Constant/1 -> Sample and Hold/Trigger, Switch/2
  Delay/1 -> Sample and Hold/1
  Sample and Hold/1 -> Switch/1
  Switch/1 -> Subsystem5/1(input [deg])

== system TOGGLER/isWFCStrategyOn? ==
  INFLW_Status : Inport
  WFCStatus : Inport  Port=2
  isAvailable : Inport  Port=3
  ManualActivation : Inport  Port=4
  Compare To Constant1 : simulink/Logic and Bit Operations/Compare To Constant  relop===  const=1  OutDataTypeStr=boolean
  Compare To Constant7 : simulink/Logic and Bit Operations/Compare To Constant  relop===  const=1  OutDataTypeStr=boolean
  Compare To Constant8 : simulink/Logic and Bit Operations/Compare To Constant  relop===  const=1  OutDataTypeStr=boolean
  Logical Operator3 : Logic  Inputs=4  AllPortsSameDT=off  OutDataTypeStr=boolean
  isActive : Outport  VectorParamsAs1DForOutWhenUnconnected=off
  wires:
  isAvailable/1 -> Logical Operator3/3
  Compare To Constant7/1 -> Logical Operator3/1
  Compare To Constant8/1 -> Logical Operator3/2
  Logical Operator3/1 -> isActive/1
  INFLW_Status/1 -> Compare To Constant7/1
  WFCStatus/1 -> Compare To Constant8/1
  ManualActivation/1 -> Compare To Constant1/1
  Compare To Constant1/1 -> Logical Operator3/4

== system TOGGLER/isWFCStrategyOn?1 ==
  INFLW_Status : Inport
  WFCStatus : Inport  Port=2
  isAvailable : Inport  Port=3
  ManualActivation : Inport  Port=4
  Compare To Constant1 : simulink/Logic and Bit Operations/Compare To Constant  relop===  const=1  OutDataTypeStr=boolean
  Compare To Constant7 : simulink/Logic and Bit Operations/Compare To Constant  relop===  const=1  OutDataTypeStr=boolean
  Compare To Constant8 : simulink/Logic and Bit Operations/Compare To Constant  relop===  const=1  OutDataTypeStr=boolean
  Logical Operator3 : Logic  Inputs=4  AllPortsSameDT=off  OutDataTypeStr=boolean
  isActive : Outport  VectorParamsAs1DForOutWhenUnconnected=off
  wires:
  ManualActivation/1 -> Compare To Constant1/1
  WFCStatus/1 -> Compare To Constant8/1
  INFLW_Status/1 -> Compare To Constant7/1
  Logical Operator3/1 -> isActive/1
  Compare To Constant8/1 -> Logical Operator3/2
  Compare To Constant7/1 -> Logical Operator3/1
  isAvailable/1 -> Logical Operator3/3
  Compare To Constant1/1 -> Logical Operator3/4

== system TOGGLER/isWFCStrategyOn?2 ==
  INFLW_Status : Inport
  WFCStatus : Inport  Port=2
  isAvailable : Inport  Port=3
  ManualActivation : Inport  Port=4
  Compare To Constant1 : simulink/Logic and Bit Operations/Compare To Constant  relop===  const=1  OutDataTypeStr=boolean
  Compare To Constant7 : simulink/Logic and Bit Operations/Compare To Constant  relop===  const=1  OutDataTypeStr=boolean
  Compare To Constant8 : simulink/Logic and Bit Operations/Compare To Constant  relop===  const=1  OutDataTypeStr=boolean
  Logical Operator3 : Logic  Inputs=4  AllPortsSameDT=off  OutDataTypeStr=boolean
  isActive : Outport  VectorParamsAs1DForOutWhenUnconnected=off
  wires:
  isAvailable/1 -> Logical Operator3/3
  Compare To Constant7/1 -> Logical Operator3/1
  Compare To Constant8/1 -> Logical Operator3/2
  Logical Operator3/1 -> isActive/1
  INFLW_Status/1 -> Compare To Constant7/1
  WFCStatus/1 -> Compare To Constant8/1
  ManualActivation/1 -> Compare To Constant1/1
  Compare To Constant1/1 -> Logical Operator3/4

== system TOGGLER/isWFCStrategyOn?3 ==
  INFLW_Status : Inport
  WFCStatus : Inport  Port=2
  isAvailable : Inport  Port=3
  ManualActivation : Inport  Port=4
  Compare To Constant1 : simulink/Logic and Bit Operations/Compare To Constant  relop===  const=1  OutDataTypeStr=boolean
  Compare To Constant7 : simulink/Logic and Bit Operations/Compare To Constant  relop===  const=1  OutDataTypeStr=boolean
  Compare To Constant8 : simulink/Logic and Bit Operations/Compare To Constant  relop===  const=1  OutDataTypeStr=boolean
  Logical Operator3 : Logic  Inputs=4  AllPortsSameDT=off  OutDataTypeStr=boolean
  isActive : Outport  VectorParamsAs1DForOutWhenUnconnected=off
  wires:
  Compare To Constant1/1 -> Logical Operator3/4
  ManualActivation/1 -> Compare To Constant1/1
  WFCStatus/1 -> Compare To Constant8/1
  INFLW_Status/1 -> Compare To Constant7/1
  Logical Operator3/1 -> isActive/1
  Compare To Constant8/1 -> Logical Operator3/2
  Compare To Constant7/1 -> Logical Operator3/1
  isAvailable/1 -> Logical Operator3/3

== system TOGGLER/Check Input/Subsystem5 ==
  InVar : Inport
  StartupTimeSamples : Inport  Port=2
  Constant : Constant  Value=0
  Delay : Delay  DelayLength=1  InitialCondition=0
  GreaterThan : RelationalOperator  Operator=>  OutDataTypeStr=boolean  RndMeth=Simplest  InputSameDT=off
  Logical Operator : Logic  Operator=OR  AllPortsSameDT=off  OutDataTypeStr=boolean
  Moving Standard Deviation1 : dspstat3/Moving Standard Deviation  Method=Sliding window  ForgettingFactorPort=off  SpecifyWindowLength=on  WindowLength=CTRL.InputCheck.MovAvErrorCheck  OverlapLength=CTRL.InputCheck.MovAvErrorCheck -1  AllowArbitraryInputLength=off  ForgettingFactor=0.9  SimulateUsing=Code generation
  One : Constant  OutDataTypeStr=Inherit: Inherit via back propagation
  Saturation Dynamic : simulink/Discontinuities/Saturation Dynamic  OutMin=[]  OutMax=[]  OutDataTypeStr=Inherit: Same as second input  OutDataType=fixdt(1, 16)  OutScaling=2^-10  DoSatur=off
  Subsystem5 : Subsystem
  Sum : Sum  Inputs=|++
  Var : Outport  VectorParamsAs1DForOutWhenUnconnected=off
  ErrorFlag : Outport  Port=2  VectorParamsAs1DForOutWhenUnconnected=off
  wires:
  Saturation Dynamic/1 -> GreaterThan/2
  Constant/1 -> Saturation Dynamic/3
  GreaterThan/1 -> Logical Operator/2
  Delay/1 -> Sum/2
  One/1 -> Sum/1
  Sum/1 -> Saturation Dynamic/2, Delay/1
  StartupTimeSamples/1 -> GreaterThan/1, Saturation Dynamic/1
  Logical Operator/1 -> ErrorFlag/1
  Subsystem5/1(ErrorFlag) -> Logical Operator/1
  Moving Standard Deviation1/1 -> Subsystem5/1(In1)
  InVar/1 -> Moving Standard Deviation1/1, Var/1

== system TOGGLER/Check Input/Subsystem6 ==
  InVar : Inport
  StartupTimeSamples : Inport  Port=2
  Constant : Constant  Value=0
  Delay : Delay  DelayLength=1  InitialCondition=0
  GreaterThan : RelationalOperator  Operator=>  OutDataTypeStr=boolean  RndMeth=Simplest  InputSameDT=off
  Logical Operator : Logic  Operator=OR  AllPortsSameDT=off  OutDataTypeStr=boolean
  Moving Standard Deviation1 : dspstat3/Moving Standard Deviation  Method=Sliding window  ForgettingFactorPort=off  SpecifyWindowLength=on  WindowLength=CTRL.InputCheck.MovAvErrorCheck  OverlapLength=CTRL.InputCheck.MovAvErrorCheck - 1  AllowArbitraryInputLength=off  ForgettingFactor=0.9  SimulateUsing=Code generation
  One : Constant  OutDataTypeStr=Inherit: Inherit via back propagation
  Saturation Dynamic : simulink/Discontinuities/Saturation Dynamic  OutMin=[]  OutMax=[]  OutDataTypeStr=Inherit: Same as second input  OutDataType=fixdt(1, 16)  OutScaling=2^-10  DoSatur=off
  Subsystem5 : Subsystem
  Sum : Sum  Inputs=|++
  Var : Outport  VectorParamsAs1DForOutWhenUnconnected=off
  ErrorFlag : Outport  Port=2  VectorParamsAs1DForOutWhenUnconnected=off
  wires:
  InVar/1 -> Var/1, Moving Standard Deviation1/1
  Moving Standard Deviation1/1 -> Subsystem5/1(In1)
  Subsystem5/1(ErrorFlag) -> Logical Operator/1
  Logical Operator/1 -> ErrorFlag/1
  StartupTimeSamples/1 -> Saturation Dynamic/1, GreaterThan/1
  Sum/1 -> Delay/1, Saturation Dynamic/2
  One/1 -> Sum/1
  Delay/1 -> Sum/2
  GreaterThan/1 -> Logical Operator/2
  Constant/1 -> Saturation Dynamic/3
  Saturation Dynamic/1 -> GreaterThan/2

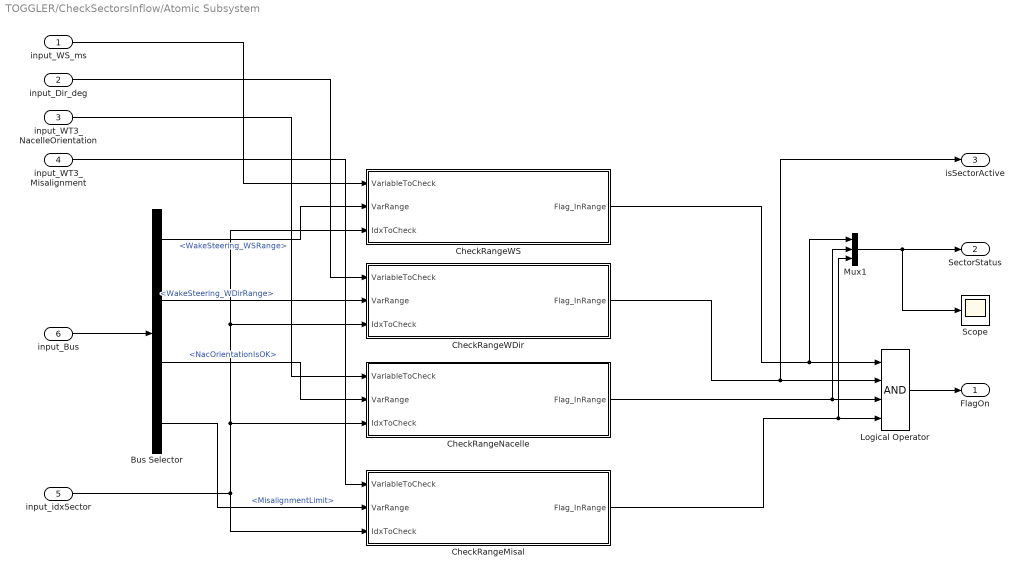
== system TOGGLER/CheckSectorsInflow/Atomic Subsystem ==
  input_WS_ms : Inport  PortDimensions=1
  input_Dir_deg : Inport  Port=2  PortDimensions=1
  input_WT3_NacelleOrientation : Inport  Port=3
  input_WT3_Misalignment : Inport  Port=4  OutDataTypeStr=double  PortDimensions=1
  input_idxSector : Inport  Port=5  OutDataTypeStr=double  PortDimensions=1
  input_Bus : Inport  Port=6  PortDimensions=1
  Bus Selector : BusSelector  OutputSignals=WakeSteering_WSRange,WakeSteering_WDirRange,NacOrientationIsOK,MisalignmentLimit
  CheckRangeMisal : Subsystem
  CheckRangeNacelle : Subsystem
  CheckRangeWDir : Subsystem
  CheckRangeWS : Subsystem
  Logical Operator : Logic  Inputs=4  AllPortsSameDT=off  OutDataTypeStr=boolean
  Mux1 : Mux  Inputs=3
  Scope : Scope
  FlagOn : Outport  VectorParamsAs1DForOutWhenUnconnected=off
  SectorStatus : Outport  Port=2  VectorParamsAs1DForOutWhenUnconnected=off
  isSectorActive : Outport  Port=3  VectorParamsAs1DForOutWhenUnconnected=off
  wires:
  CheckRangeWS/1(Flag_InRange) -> Mux1/1, Logical Operator/1
  input_Bus/1 -> Bus Selector/1
  Bus Selector/2 -> CheckRangeWDir/2(VarRange)  "<WakeSteering_WDirRange>"
  Bus Selector/3 -> CheckRangeNacelle/2(VarRange)  "<NacOrientationIsOK>"
  Bus Selector/4 -> CheckRangeMisal/2(VarRange)  "<MisalignmentLimit>"
  input_idxSector/1 -> CheckRangeWS/3(IdxToCheck), CheckRangeWDir/3(IdxToCheck), CheckRangeNacelle/3(IdxToCheck), CheckRangeMisal/3(IdxToCheck)
  input_WS_ms/1 -> CheckRangeWS/1(VariableToCheck)
  Bus Selector/1 -> CheckRangeWS/2(VarRange)  "<WakeSteering_WSRange>"
  input_Dir_deg/1 -> CheckRangeWDir/1(VariableToCheck)
  input_WT3_NacelleOrientation/1 -> CheckRangeNacelle/1(VariableToCheck)
  CheckRangeNacelle/1(Flag_InRange) -> Mux1/2, Logical Operator/3
  input_WT3_Misalignment/1 -> CheckRangeMisal/1(VariableToCheck)
  CheckRangeWDir/1(Flag_InRange) -> isSectorActive/1, Logical Operator/2
  CheckRangeMisal/1(Flag_InRange) -> Mux1/3, Logical Operator/4
  Logical Operator/1 -> FlagOn/1
  Mux1/1 -> SectorStatus/1, Scope/1

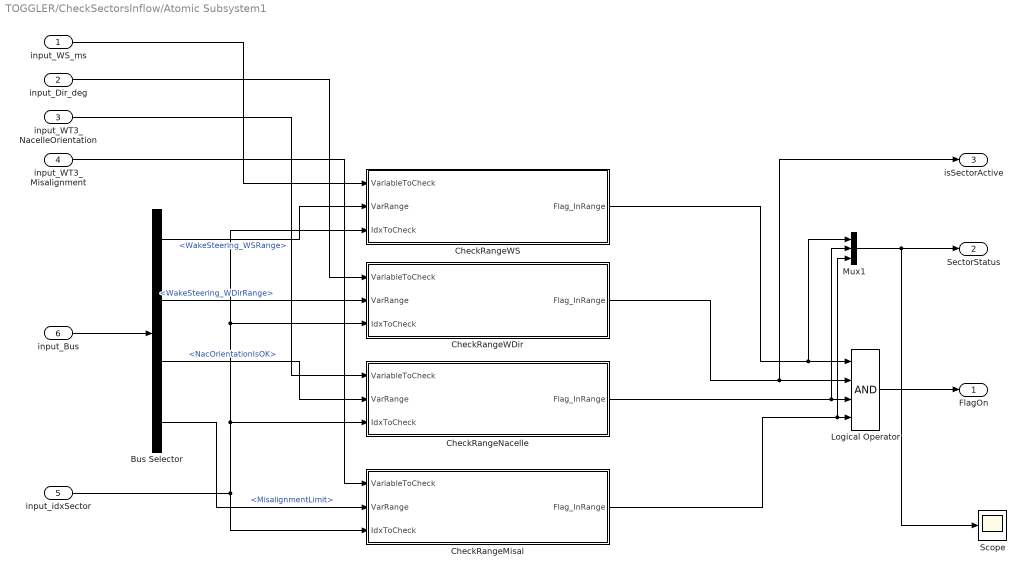
== system TOGGLER/CheckSectorsInflow/Atomic Subsystem1 ==
  input_WS_ms : Inport  PortDimensions=1
  input_Dir_deg : Inport  Port=2  PortDimensions=1
  input_WT3_NacelleOrientation : Inport  Port=3
  input_WT3_Misalignment : Inport  Port=4  OutDataTypeStr=double  PortDimensions=1
  input_idxSector : Inport  Port=5  OutDataTypeStr=double  PortDimensions=1
  input_Bus : Inport  Port=6  PortDimensions=1
  Bus Selector : BusSelector  OutputSignals=WakeSteering_WSRange,WakeSteering_WDirRange,NacOrientationIsOK,MisalignmentLimit
  CheckRangeMisal : Subsystem
  CheckRangeNacelle : Subsystem
  CheckRangeWDir : Subsystem
  CheckRangeWS : Subsystem
  Logical Operator : Logic  Inputs=4  AllPortsSameDT=off  OutDataTypeStr=boolean
  Mux1 : Mux  Inputs=3
  Scope : Scope
  FlagOn : Outport  VectorParamsAs1DForOutWhenUnconnected=off
  SectorStatus : Outport  Port=2  VectorParamsAs1DForOutWhenUnconnected=off
  isSectorActive : Outport  Port=3  VectorParamsAs1DForOutWhenUnconnected=off
  wires:
  Mux1/1 -> Scope/1, SectorStatus/1
  Logical Operator/1 -> FlagOn/1
  CheckRangeMisal/1(Flag_InRange) -> Logical Operator/4, Mux1/3
  CheckRangeWDir/1(Flag_InRange) -> Logical Operator/2, isSectorActive/1
  input_WT3_Misalignment/1 -> CheckRangeMisal/1(VariableToCheck)
  CheckRangeNacelle/1(Flag_InRange) -> Logical Operator/3, Mux1/2
  input_WT3_NacelleOrientation/1 -> CheckRangeNacelle/1(VariableToCheck)
  input_Dir_deg/1 -> CheckRangeWDir/1(VariableToCheck)
  Bus Selector/1 -> CheckRangeWS/2(VarRange)  "<WakeSteering_WSRange>"
  input_WS_ms/1 -> CheckRangeWS/1(VariableToCheck)
  input_idxSector/1 -> CheckRangeMisal/3(IdxToCheck), CheckRangeNacelle/3(IdxToCheck), CheckRangeWDir/3(IdxToCheck), CheckRangeWS/3(IdxToCheck)
  Bus Selector/4 -> CheckRangeMisal/2(VarRange)  "<MisalignmentLimit>"
  Bus Selector/3 -> CheckRangeNacelle/2(VarRange)  "<NacOrientationIsOK>"
  Bus Selector/2 -> CheckRangeWDir/2(VarRange)  "<WakeSteering_WDirRange>"
  input_Bus/1 -> Bus Selector/1
  CheckRangeWS/1(Flag_InRange) -> Logical Operator/1, Mux1/1

== system TOGGLER/Subsystem2/Enabled Subsystem ==
  In1 : Inport
  Enable : EnablePort
  Out1 : Outport  VectorParamsAs1DForOutWhenUnconnected=off
  wires:
  In1/1 -> Out1/1

== system TOGGLER/Subsystem2/Enabled Subsystem1 ==
  In1 : Inport
  Enable : EnablePort
  Out1 : Outport  VectorParamsAs1DForOutWhenUnconnected=off
  wires:
  In1/1 -> Out1/1

== system TOGGLER/Subsystem3/Enabled Subsystem ==
  In1 : Inport
  Enable : EnablePort
  Out1 : Outport  VectorParamsAs1DForOutWhenUnconnected=off
  wires:
  In1/1 -> Out1/1

== system TOGGLER/Subsystem3/Enabled Subsystem1 ==
  In1 : Inport
  Enable : EnablePort
  Out1 : Outport  VectorParamsAs1DForOutWhenUnconnected=off
  wires:
  In1/1 -> Out1/1

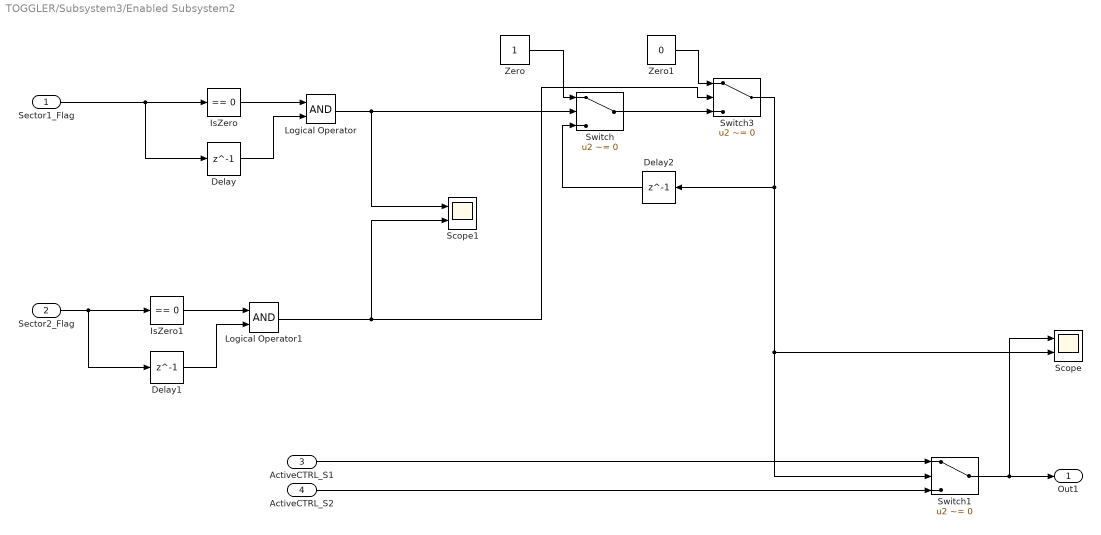
== system TOGGLER/Subsystem3/Enabled Subsystem2 ==
  Sector1_Flag : Inport
  Sector2_Flag : Inport  Port=2
  ActiveCTRL_S1 : Inport  Port=3
  ActiveCTRL_S2 : Inport  Port=4
  Delay : Delay  DelayLength=1  InitialCondition=0
  Delay1 : Delay  DelayLength=1  InitialCondition=0
  Delay2 : Delay  DelayLength=1  InitialCondition=0
  IsZero : simulink/Logic and Bit Operations/Compare To Zero  relop===  OutDataTypeStr=boolean
  IsZero1 : simulink/Logic and Bit Operations/Compare To Zero  relop===  OutDataTypeStr=boolean
  Logical Operator : Logic  AllPortsSameDT=off  OutDataTypeStr=boolean
  Logical Operator1 : Logic  AllPortsSameDT=off  OutDataTypeStr=boolean
  Scope : Scope  NumInputPorts=2
  Scope1 : Scope  NumInputPorts=2
  Switch : Switch  Criteria=u2 ~= 0  SaturateOnIntegerOverflow=off  InputSameDT=off
  Switch1 : Switch  Criteria=u2 ~= 0  SaturateOnIntegerOverflow=off  InputSameDT=off
  Switch3 : Switch  Criteria=u2 ~= 0  SaturateOnIntegerOverflow=off  InputSameDT=off
  Zero : Constant  OutDataTypeStr=Inherit: Inherit via back propagation
  Zero1 : Constant  Value=0  OutDataTypeStr=Inherit: Inherit via back propagation
  Out1 : Outport  VectorParamsAs1DForOutWhenUnconnected=off
  wires:
  Sector1_Flag/1 -> IsZero/1, Delay/1
  Delay/1 -> Logical Operator/2
  IsZero/1 -> Logical Operator/1
  IsZero1/1 -> Logical Operator1/1
  Delay1/1 -> Logical Operator1/2
  Sector2_Flag/1 -> Delay1/1, IsZero1/1
  ActiveCTRL_S1/1 -> Switch1/1
  Logical Operator/1 -> Scope1/1, Switch/2
  ActiveCTRL_S2/1 -> Switch1/3
  Switch1/1 -> Scope/1, Out1/1
  Switch/1 -> Switch3/3
  Delay2/1 -> Switch/3
  Logical Operator1/1 -> Scope1/2, Switch3/2
  Zero/1 -> Switch/1
  Zero1/1 -> Switch3/1
  Switch3/1 -> Switch1/2, Scope/2, Delay2/1

== system TOGGLER/Subsystem3/Enabled Subsystem3 ==
  In1 : Inport
  Enable : EnablePort
  Out1 : Outport  VectorParamsAs1DForOutWhenUnconnected=off
  wires:
  In1/1 -> Out1/1

== system TOGGLER/Subsystem3/Subsystem ==
  Sect1 : Inport
  XOR : Inport  Port=2
  Sect2 : Inport  Port=3
  Logical Operator : Logic  AllPortsSameDT=off  OutDataTypeStr=boolean
  Logical Operator1 : Logic  AllPortsSameDT=off  OutDataTypeStr=boolean
  NOT : Logic  Operator=NOT  IconShape=distinctive  AllPortsSameDT=off  OutDataTypeStr=boolean
  Sector1_Flag : Outport  VectorParamsAs1DForOutWhenUnconnected=off
  Sector2_Flag : Outport  Port=2  VectorParamsAs1DForOutWhenUnconnected=off
  Off : Outport  Port=3  VectorParamsAs1DForOutWhenUnconnected=off
  wires:
  Logical Operator1/1 -> Sector2_Flag/1
  Sect2/1 -> Logical Operator1/1
  XOR/1 -> Logical Operator/2, Logical Operator1/2, NOT/1
  Logical Operator/1 -> Sector1_Flag/1
  Sect1/1 -> Logical Operator/1
  NOT/1 -> Off/1

== system TOGGLER/Subsystem4/Subsystem ==
  FlagTurbineWFCIsOn : Inport
  AvailableCTRL : Inport  Port=2
  FlagWFCIsActive : Inport  Port=3
  CTRLList : Inport  Port=4
  TogglingSamples : Inport  Port=5
  Memory1 : Memory
  Memory2 : Memory
  Toggler : MATLAB Function  TreatAsAtomicUnit=on
  WFC Time Manager : Subsystem  mask(WFC Time manager){sample_time=sample_time, TimeManagFlag=CTRL.AutomTimeMGMT.ActivFlag, TriggerTime=CTRL.AutomTimeMGMT.TriggerTime, ReductionFactor=CTRL.AutomTimeMGMT.ReductionFactor}
      mask prompts: sample_time "Sampling time [s]"; TimeManagFlag "Automatic time redistribution Flag [0/1]"; TriggerTime "Redistribution trigger time [Hrs]"; ReductionFactor "Reduction Factor [-]"
      mask help:
      | This function monitors the execution time of each WFC strategy and gives as output the time for which each control strategy was active on the turbine.
      | The option "Automatic time redistribution" allows the user to give priority to those strategy tha have run for a shorter amount of time, specified by the "Redistribution trigger time" field. If this option is enabled, a strategy whose deviation exceeds "Redistribution trigger time" from the mean of all the active strategies, will be skipped until its deviation is reduced by a factor specified by "Reduction Factor"
      mask Help: Ask Carlo Sucameli for help
      mask Callback TimeManagFlag:
      | TMF = get_param(gcb,'TimeManagFlag');
      | m = Simulink.Mask.get(gcb);
      | TT = m.getParameter('TriggerTime');
      | 
      | if strcmp(TMF,'1')
      |   TT.Enabled = 'on';
      | else
      |    TT.Enabled = 'off';
      | end
      | 
      | RF = m.getParameter('ReductionFactor');
      | 
      | if strcmp(TMF,'1')
      |   RF.Enabled = 'on';
      | else
      |    RF.Enabled = 'off';
      | end
  onTime_Hrs : Outport  VectorParamsAs1DForOutWhenUnconnected=off
  tot_OnTime_Hrs : Outport  Port=2  VectorParamsAs1DForOutWhenUnconnected=off
  ActiveCTRL : Outport  Port=3  VectorParamsAs1DForOutWhenUnconnected=off
  wires:
  WFC Time Manager/3(Updated_Counter) -> Memory1/1
  WFC Time Manager/1(tot_OnTime_Hrs) -> tot_OnTime_Hrs/1
  AvailableCTRL/1 -> Toggler/1(AvailableCTRL), WFC Time Manager/5(AvailableCTRL)
  CTRLList/1 -> WFC Time Manager/4(CTRLList), Toggler/2(CTRLList)
  Memory2/1 -> Toggler/3(OldActiveCTRL)
  WFC Time Manager/2(onTime_Hrs) -> onTime_Hrs/1
  Memory1/1 -> Toggler/4(OldCounter)
  Toggler/2(Counter) -> WFC Time Manager/6(Counter)
  FlagTurbineWFCIsOn/1 -> WFC Time Manager/1(Flag_TurbineWFCIsActive)
  Toggler/1(ActiveCTRL) -> ActiveCTRL/1, Memory2/1, WFC Time Manager/3(ActiveCTRL)
  FlagWFCIsActive/1 -> WFC Time Manager/2(Flag_WFCIsActive)
  TogglingSamples/1 -> Toggler/5(TogglingSamples)

== system TOGGLER/Subsystem4/Subsystem1 ==
  Sect1 : Inport
  XOR : Inport  Port=2
  Sect2 : Inport  Port=3
  Logical Operator : Logic  AllPortsSameDT=off  OutDataTypeStr=boolean
  Logical Operator1 : Logic  AllPortsSameDT=off  OutDataTypeStr=boolean
  NOT : Logic  Operator=NOT  IconShape=distinctive  AllPortsSameDT=off  OutDataTypeStr=boolean
  Sector1_Flag : Outport  VectorParamsAs1DForOutWhenUnconnected=off
  Sector2_Flag : Outport  Port=2  VectorParamsAs1DForOutWhenUnconnected=off
  Off : Outport  Port=3  VectorParamsAs1DForOutWhenUnconnected=off
  wires:
  Logical Operator1/1 -> Sector2_Flag/1
  Sect2/1 -> Logical Operator1/1
  XOR/1 -> Logical Operator/2, Logical Operator1/2, NOT/1
  Logical Operator/1 -> Sector1_Flag/1
  Sect1/1 -> Logical Operator/1
  NOT/1 -> Off/1

== system TOGGLER/Subsystem4/Subsystem3 ==
  FlagTurbineWFCIsOn : Inport
  AvailableCTRL : Inport  Port=2
  FlagWFCIsActive : Inport  Port=3
  CTRLList : Inport  Port=4
  TogglingSamples : Inport  Port=5
  Memory1 : Memory
  Memory2 : Memory
  Toggler : MATLAB Function  TreatAsAtomicUnit=on
  WFC Time Manager : Subsystem  mask(WFC Time manager){sample_time=sample_time, TimeManagFlag=CTRL.AutomTimeMGMT.ActivFlag, TriggerTime=CTRL.AutomTimeMGMT.TriggerTime, ReductionFactor=CTRL.AutomTimeMGMT.ReductionFactor}
      mask prompts: sample_time "Sampling time [s]"; TimeManagFlag "Automatic time redistribution Flag [0/1]"; TriggerTime "Redistribution trigger time [Hrs]"; ReductionFactor "Reduction Factor [-]"
      mask help:
      | This function monitors the execution time of each WFC strategy and gives as output the time for which each control strategy was active on the turbine.
      | The option "Automatic time redistribution" allows the user to give priority to those strategy tha have run for a shorter amount of time, specified by the "Redistribution trigger time" field. If this option is enabled, a strategy whose deviation exceeds "Redistribution trigger time" from the mean of all the active strategies, will be skipped until its deviation is reduced by a factor specified by "Reduction Factor"
      mask Help: Ask Carlo Sucameli for help
      mask Callback TimeManagFlag:
      | TMF = get_param(gcb,'TimeManagFlag');
      | m = Simulink.Mask.get(gcb);
      | TT = m.getParameter('TriggerTime');
      | 
      | if strcmp(TMF,'1')
      |   TT.Enabled = 'on';
      | else
      |    TT.Enabled = 'off';
      | end
      | 
      | RF = m.getParameter('ReductionFactor');
      | 
      | if strcmp(TMF,'1')
      |   RF.Enabled = 'on';
      | else
      |    RF.Enabled = 'off';
      | end
  onTime_Hrs : Outport  VectorParamsAs1DForOutWhenUnconnected=off
  tot_OnTime_Hrs : Outport  Port=2  VectorParamsAs1DForOutWhenUnconnected=off
  ActiveCTRL : Outport  Port=3  VectorParamsAs1DForOutWhenUnconnected=off
  wires:
  TogglingSamples/1 -> Toggler/5(TogglingSamples)
  FlagWFCIsActive/1 -> WFC Time Manager/2(Flag_WFCIsActive)
  Toggler/1(ActiveCTRL) -> WFC Time Manager/3(ActiveCTRL), Memory2/1, ActiveCTRL/1
  FlagTurbineWFCIsOn/1 -> WFC Time Manager/1(Flag_TurbineWFCIsActive)
  Toggler/2(Counter) -> WFC Time Manager/6(Counter)
  Memory1/1 -> Toggler/4(OldCounter)
  WFC Time Manager/2(onTime_Hrs) -> onTime_Hrs/1
  Memory2/1 -> Toggler/3(OldActiveCTRL)
  CTRLList/1 -> Toggler/2(CTRLList), WFC Time Manager/4(CTRLList)
  AvailableCTRL/1 -> WFC Time Manager/5(AvailableCTRL), Toggler/1(AvailableCTRL)
  WFC Time Manager/1(tot_OnTime_Hrs) -> tot_OnTime_Hrs/1
  WFC Time Manager/3(Updated_Counter) -> Memory1/1
